simulink model "passthrough"  (R2023b)
settings: Solver=FixedStepDiscrete  StartTime=0.0  StopTime=inf  FixedStep=1/100  RelTol=1e-3
undefined symbols (not defined in the file): DiscIntNeverNeededParam
settings Model: Creator=asd  LastModifiedBy=asd
settings SolverCC: InsertRTBMode=Always
settings DataIOCC: ExternalInput=dt  InitialState=[dt]
settings OptimizationCC: DefaultParameterBehavior=Inlined  DefaultUnderspecifiedDataType=single  EnhancedBackFolding=on  PassReuseOutputArgsAs=Individual arguments  ZeroExternalMemoryAtStartup=off  ZeroInternalMemoryAtStartup=off  RemoveLocalVariableInitialization=off  OptimizeBlockOrder=speed  DifferentSizesBufferReuse=on  OptimizationCustomize=off  LabelGuidedReuse=on  EfficientTunableParamExpr=on
settings DebuggingCC: ParameterTunabilityLossMsg=error
settings HardwareCC: ProdBitPerPointer=32  ProdBitPerSizeT=32  ProdBitPerPtrDiffT=32  ProdLargestAtomicInteger=Long  ProdLargestAtomicFloat=Double  ProdWordSize=32  ProdHWDeviceType=ARM Compatible->ARM Cortex-M
settings SFSimCC: MATLABDynamicMemAlloc=off
settings RTWCC: Description=Embedded Coder  SystemTargetFile=ert.tlc  GenCodeOnly=on  TemplateMakefile=ert_default_tmf  CustomSourceCode="#pragma GCC diagnostic ignored \"-Wfloat-equal\""  DataTypeReplacement=CDataTypesFixedWidth  TargetLang=C++
settings CodeAppCC: ForceParamTrailComments=on  IgnoreCustomStorageClasses=off  OperatorAnnotations=on  SimulinkDataObjDesc=on  SFDataObjDesc=on  CustomSymbolStrGlobalVar=$N$M  CustomSymbolStrType=$N$M_T  CustomSymbolStrFcn=$N$M$F  CustomSymbolStrMacro=$N$M  InsertBlockDesc=on  InlinedPrmAccess=Macros
settings ERTTargetCC: TargetLangStandard=C++11 (ISO)  GenerateSampleERTMain=on  CombineSignalStateStructs=on  GroupInternalDataByFunction=on  SuppressErrorStatus=on  CodeInterfacePackaging=C++ class  SupportComplex=off  RemoveResetFunc=off  DSAsUniqueAccess=on  ExtModeTransport=2  ExtModeStaticAlloc=on  ExtModeMaxTrigDuration=1000000  ExtModeMexFile=ext_xcp  ExtModeIntrfLevel=Level2 - Open  RootIOFormat=Structure reference  ERTCustomFileTemplate=example_file_process.tlc  ERTFilePackagingFormat=Compact  MaxIdInt64=INT64_MAX  MinIdInt64=INT64_MIN  MaxIdUint64=UINT64_MAX  MaxIdInt32=INT32_MAX  MinIdInt32=INT32_MIN  MaxIdUint32=UINT32_MAX  MaxIdInt16=INT16_MAX  MinIdInt16=INT16_MIN  MaxIdUint16=UINT16_MAX  MaxIdInt8=INT8_MAX  MinIdInt8=INT8_MIN  MaxIdUint8=UINT8_MAX

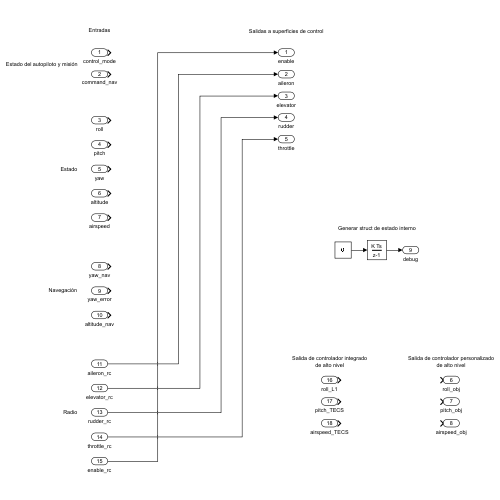
[thumbnail: Simulink's stored preview of the top-level diagram]
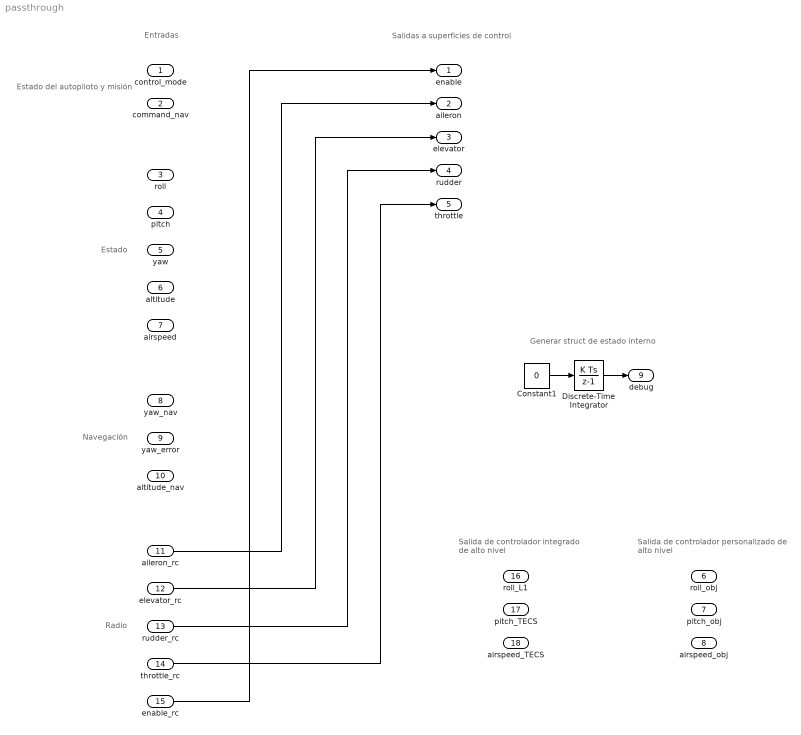
== system passthrough ==
  note: Generar struct de estado interno
  note: Salidas a superficies de control
  note: Salida de controlador personalizado
      | de alto nivel
  note: Salida de controlador integrado
      | de alto nivel
  note: Radio
  note: Navegación
  note: Estado
  note: Estado del autopiloto y misión
  note: Entradas
  control_mode : Inport  OutDataTypeStr=single
  command_nav : Inport  Port=2
  roll : Inport  Port=3
  pitch : Inport  Port=4
  yaw : Inport  Port=5
  altitude : Inport  Port=6
  airspeed : Inport  Port=7  OutDataTypeStr=single
  yaw_nav : Inport  Port=8
  yaw_error : Inport  Port=9
  altitude_nav : Inport  Port=10
  aileron_rc : Inport  Port=11
  elevator_rc : Inport  Port=12
  rudder_rc : Inport  Port=13
  throttle_rc : Inport  Port=14  OutDataTypeStr=single
  enable_rc : Inport  Port=15  OutDataTypeStr=boolean
  roll_L1 : Inport  Port=16
  pitch_TECS : Inport  Port=17
  airspeed_TECS : Inport  Port=18
  Constant1 : Constant  Value=0  OutDataTypeStr=single
  Discrete-Time Integrator : DiscreteIntegrator  SampleTime=-1  ICPrevOutput=DiscIntNeverNeededParam  ICPrevScaledInput=DiscIntNeverNeededParam
  enable : Outport  OutDataTypeStr=boolean
  aileron : Outport  Port=2
  elevator : Outport  Port=3
  rudder : Outport  Port=4
  throttle : Outport  Port=5  OutDataTypeStr=single
  roll_obj : Outport  Port=6
  pitch_obj : Outport  Port=7
  airspeed_obj : Outport  Port=8  OutDataTypeStr=single
  debug : Outport  Port=9
  wires:
  aileron_rc/1 -> aileron/1
  elevator_rc/1 -> elevator/1
  rudder_rc/1 -> rudder/1
  throttle_rc/1 -> throttle/1
  Constant1/1 -> Discrete-Time Integrator/1
  Discrete-Time Integrator/1 -> debug/1
  enable_rc/1 -> enable/1
